simulink model "filters"  (R2024b)
settings: Solver=FixedStepDiscrete  StartTime=0.0  StopTime=10  RelTol=1e-3
libraries: dspadpt3 x2
settings Model: Creator=Mayur  LastModifiedBy=Mayur

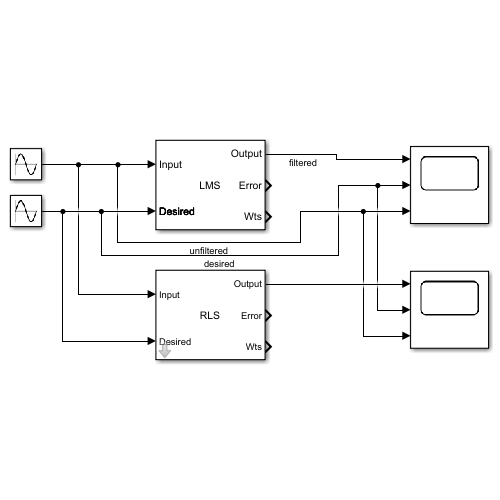
[thumbnail: Simulink's stored preview of the top-level diagram]
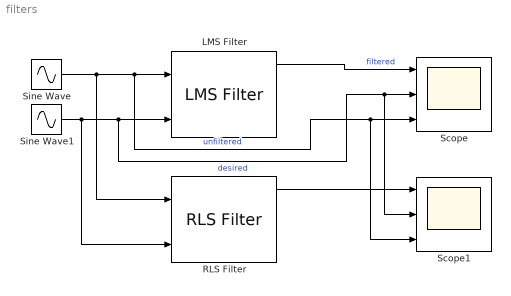
== system filters ==
  LMS Filter : dspadpt3/LMS Filter  Algo=LMS  L=32  stepflag=Dialog  mu=0.1  leakage=1.0  ic=0  Adapt=off  resetflag=None  weights=on  addnparflag=off  roundingMode=Floor  overflowMode=off
  RLS Filter : dspadpt3/RLS Filter  L=32  lambdaflag=Dialog  lambda=1  addnparflag=on  ic=0  delta=0.1  Adapt=off  resetflag=None  weights=on
  Scope : Scope  NumInputPorts=3
  Scope1 : Scope  NumInputPorts=3
  Sine Wave : Sin  SampleTime=0
  Sine Wave1 : Sin  Phase=10  SampleTime=0
  wires:
  Sine Wave1/1 -> RLS Filter/2, Scope1/2, Scope/2, LMS Filter/2  "desired"
  LMS Filter/1 -> Scope/1  "filtered"
  Sine Wave/1 -> RLS Filter/1, Scope1/3, Scope/3, LMS Filter/1  "unfiltered"
  RLS Filter/1 -> Scope1/1
